simulink model "Eem_StMac_Prj"  (R2013b)
settings: Solver=FixedStepDiscrete  StartTime=0.0  StopTime=inf  FixedStep=0.001  RelTol=1e-3
PreLoadFcn:
  | load('Eem_StMac_Sim_DataSpec.mat')
model workspace (MAT data in the model file):
  cfg_mdx : org.apache.xerces.dom.DocumentImpl (value not decoded)
  cfg_mdx_status = ASAM_PSP.MDX.Config.ConfigStatus
undefined symbols (not defined in the file): process, ProcessTrigger_Lib
libraries: Variable_Lib x21, Efx_Library x17, Parameter_Lib x16, DSM_Library x9, DeltaTime_Lib x2, SYC_Library x1, DGS_Misc_Lib x1
(part 1 of 2)
PreSaveFcn:
  | %BOSCHToolsStart
  | if exist('saveWorkspaceToMatFile','file')
  | saveWorkspaceToMatFile(bdroot);
  | end;
  | %BOSCHToolsEnd
settings Model: NumberOfSteps=100  Creator=gjg2si  LastModifiedBy=bij2si
settings DataIOCC: SaveFormat=StructureWithTime  SignalLoggingSaveFormat=ModelDataLogs  SaveOutput=off  SignalLogging=off  DSMLogging=off  SaveTime=off
settings OptimizationCC: InlineParams=on  UseIntDivNetSlope=on  UseFloatMulNetSlope=on  DefaultUnderspecifiedDataType=single  InlineInvariantSignals=on  EnhancedBackFolding=on  StrengthReduction=on  EnableMemcpy=off  PassReuseOutputArgsAs=Individual arguments  ExpressionDepthLimit=2147483647  ZeroExternalMemoryAtStartup=off  ZeroInternalMemoryAtStartup=off  InitFltsAndDblsToZero=on  EfficientFloat2IntCast=on  OptimizeModelRefInitCode=on  SimCompilerOptimization=On  AccelVerboseBuild=on
settings DebuggingCC: ConsistencyChecking=error  SignalInfNanChecking=warning  SignalRangeChecking=error  AlgebraicLoopMsg=error  UnderspecifiedInitializationDetection=Simplified  BlockPriorityViolationMsg=error  MinStepSizeMsg=error  SolverPrmCheckMsg=error  InheritedTsInSrcMsg=none  DiscreteInheritContinuousMsg=error  MultiTaskDSMMsg=warning  TasksWithSamePriorityMsg=error  SigSpecEnsureSampleTimeMsg=error  CheckMatrixSingularityMsg=error  ParameterUnderflowMsg=error  ParameterTunabilityLossMsg=error  FixptConstUnderflowMsg=error  FixptConstOverflowMsg=error  FixptConstPrecisionLossMsg=warning  UnnecessaryDatatypeConvMsg=warning  VectorMatrixConversionMsg=error  SignalLabelMismatchMsg=warning  UnconnectedLineMsg=error  SFcnCompatibilityMsg=warning  UniqueDataStoreMsg=error  RootOutportRequireBusObject=error  ModelReferenceIOMsg=error  ModelReferenceVersionMismatchMessage=warning  ModelReferenceIOMismatchMessage=warning  UnknownTsInhSupMsg=error  StateNameClashWarn=warning  SimStateInterfaceChecksumMismatchMsg=error  StrictBusMsg=ErrorOnBusTreatedAsVector  BusNameAdapt=ErrorWithoutRepair  NonBusSignalsTreatedAsBus=error  SFUnexpectedBacktrackingDiag=error  SFInvalidInputDataAccessInChartInitDiag=error  SFNoUnconditionalDefaultTransitionDiag=error  SFUnconditionalTransitionShadowingDiag=error
settings HardwareCC: ProdIntDivRoundTo=Zero  ProdHWDeviceType=Generic->32-bit Embedded Processor
settings ModelReferenceCC: ModelReferenceNumInstancesAllowed=Single
settings RTWCC: SystemTargetFile=mdxtarget.tlc  GenCodeOnly=on  GenerateMakefile=off  TemplateMakefile=mdxtarget.tmf  Description=Bosch MDX Target  GenerateReport=on  ProcessScript=mdxtarget_make_rtw_hook  IncludeHyperlinkInReport=on  LaunchReport=on  GenerateTraceInfo=on  GenerateTraceReport=on  GenerateTraceReportSl=on  GenerateTraceReportSf=on  GenerateTraceReportEml=on  RTWCompilerOptimization=On
settings CodeAppCC: ForceParamTrailComments=on  IgnoreCustomStorageClasses=off  IgnoreTestpoints=on  MaxIdLength=60  SFDataObjDesc=on  MangleLength=3  CustomSymbolStrField=$N$M_$A  CustomSymbolStrFcnArg=arg$I$N$M  CustomSymbolStrBlkIO=_tb_$A_$M  CustomSymbolStrTmpVar=_t_$A_$M  InsertBlockDesc=on  MATLABSourceComments=on
settings STFCustomTargetCC: CodeReplacementLibrary=AUTOSAR 4.0  UtilityFuncGeneration=Shared location  ERTMultiwordTypeDef=User defined  ERTMultiwordLength=0  IncludeMdlTerminateFcn=off  CombineOutputUpdateFcns=on  SuppressErrorStatus=on  ERTCustomFileBanners=on  SupportAbsoluteTime=off  SupportNonFinite=off  SupportComplex=off  SupportContinuousTime=off  SupportNonInlinedSFcns=off  ParenthesesLevel=Maximum  MATLABClassNameForMDSCustomization=Simulink.SoftwareTarget.ERTCustomization  GRTInterface=off  SystemTargetFile=mdxtarget.tlc
settings ERTTargetCC: CodeReplacementLibrary=AUTOSAR 4.0  UtilityFuncGeneration=Shared location  ERTMultiwordTypeDef=User defined  ERTMultiwordLength=0  ParMdlRefBuildCompliant=off  CompOptLevelCompliant=off  ConcurrentExecutionCompliant=off  IncludeMdlTerminateFcn=off  SuppressErrorStatus=on  ERTFirstTimeCompliant=off  SupportAbsoluteTime=off  SupportNonFinite=off  SupportComplex=off  ParenthesesLevel=Maximum  ModelStepFunctionPrototypeControlCompliant=off  CPPClassGenCompliant=off  GenerateASAP2=on  InlinedParameterPlacement=NonHierarchical  ERTSrcFileBannerTemplate=bosch_mdx_template.cgt  ERTHdrFileBannerTemplate=bosch_h_template.cgt  ERTCustomFileTemplate=mdx_file_process.tlc  ERTFilePackagingFormat=Compact  PreserveExpressionOrder=on  PreserveIfCondition=on  PreserveExternInFcnDecls=off

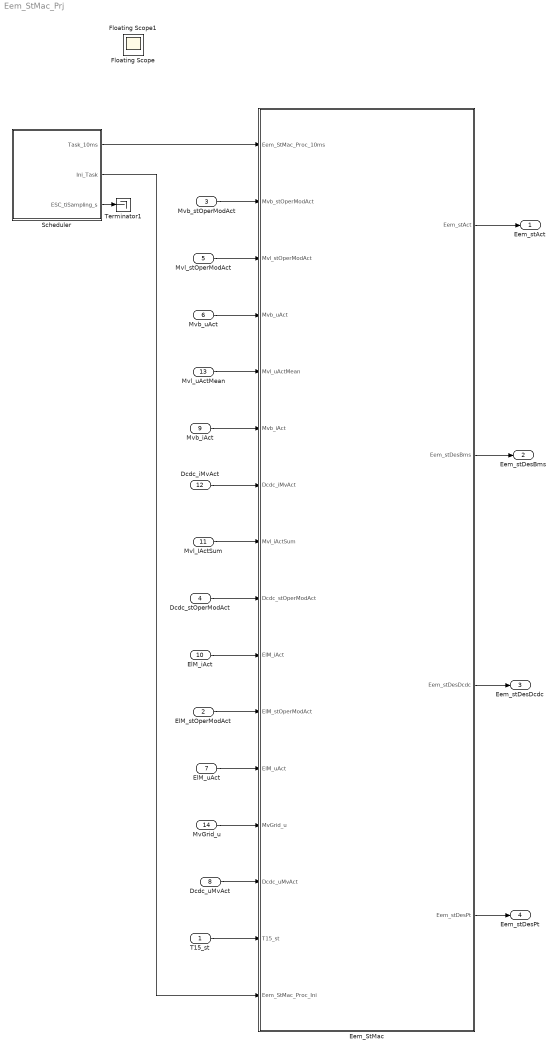
== system Eem_StMac_Prj ==
  T15_st : Inport  OutDataTypeStr=boolean
  ElM_stOperModAct : Inport  Port=2  OutDataTypeStr=OneToOne_U8
  Mvb_stOperModAct : Inport  Port=3  OutDataTypeStr=OneToOne_U8
  Dcdc_stOperModAct : Inport  Port=4  OutDataTypeStr=OneToOne_U8
  Mvl_stOperModAct : Inport  Port=5  OutDataTypeStr=OneToOne_U8
  Mvb_uAct : Inport  Port=6  OutDataTypeStr=spg_q0p0039_S16
  ElM_uAct : Inport  Port=7  OutDataTypeStr=spg_q0p0039_S16
  Dcdc_uMvAct : Inport  Port=8  OutDataTypeStr=spg_q0p0039_S16
  Mvb_iAct : Inport  Port=9  OutDataTypeStr=Curr_A_q0p03125_COMPU_S16
  ElM_iAct : Inport  Port=10  OutDataTypeStr=Curr_A_q0p03125_COMPU_S16
  Mvl_IActSum : Inport  Port=11  OutDataTypeStr=Curr_A_q0p03125_COMPU_S16
  Dcdc_iMvAct : Inport  Port=12  OutDataTypeStr=Curr_A_q0p03125_COMPU_S16
  Mvl_uActMean : Inport  Port=13  OutDataTypeStr=spg_q0p0039_S16
  MvGrid_u : Inport  Port=14  OutDataTypeStr=spg_q0p0039_S16
  Eem_StMac : Subsystem
  Scheduler : Subsystem  mask(Scheduler){Task_1ms=off, Task_2ms=off, Task_5ms=off, Task_10ms=on, Task_20ms=off, Task_50ms=off, Task_100ms=off, Task_200ms=off, Task_1000ms=off, Ini_Task=on, ASync_Task=off}
      mask help:
      | This Scheduler can be used to simulate execution of different
      | runnables/processes. Needed tasks can be de-/activated by this mask.
      |
      | Beside different time rates there is one task for initialization and
      | an asynchonous task that is triggered depending on ASync_U.
      mask init:
      | scheduler_cb('Ini',gcs,gcb);
  Terminator1 : Terminator
  Eem_stAct : Outport  OutDataTypeStr=OneToOne_U16
  Eem_stDesBms : Outport  Port=2  OutDataTypeStr=OneToOne_U8
  Eem_stDesDcdc : Outport  Port=3  OutDataTypeStr=OneToOne_U8
  Eem_stDesPt : Outport  Port=4  OutDataTypeStr=OneToOne_U8
  Floating Scope : Scope
      settings: Floating=on  YMin=0  YMax=700
  Floating Scope1 : Scope
      settings: Floating=on  YMin=0  YMax=2000
  wires:
  Scheduler/3(ESC_tiSampling_s) -> Terminator1/1
  Mvb_stOperModAct/1 -> Eem_StMac/2(Mvb_stOperModAct)
  Dcdc_stOperModAct/1 -> Eem_StMac/9(Dcdc_stOperModAct)
  Mvb_uAct/1 -> Eem_StMac/4(Mvb_uAct)
  Mvl_uActMean/1 -> Eem_StMac/5(Mvl_uActMean)
  Mvb_iAct/1 -> Eem_StMac/6(Mvb_iAct)
  Dcdc_iMvAct/1 -> Eem_StMac/7(Dcdc_iMvAct)
  Mvl_IActSum/1 -> Eem_StMac/8(Mvl_iActSum)
  Eem_StMac/1(Eem_stAct) -> Eem_stAct/1
  Eem_StMac/2(Eem_stDesBms) -> Eem_stDesBms/1
  Eem_StMac/4(Eem_stDesPt) -> Eem_stDesPt/1
  Eem_StMac/3(Eem_stDesDcdc) -> Eem_stDesDcdc/1
  Mvl_stOperModAct/1 -> Eem_StMac/3(Mvl_stOperModAct)
  Scheduler/1(Task_10ms) -> Eem_StMac/1(Eem_StMac_Proc_10ms)
  ElM_stOperModAct/1 -> Eem_StMac/11(ElM_stOperModAct)
  ElM_iAct/1 -> Eem_StMac/10(ElM_iAct)
  ElM_uAct/1 -> Eem_StMac/12(ElM_uAct)
  MvGrid_u/1 -> Eem_StMac/13(MvGrid_u)
  T15_st/1 -> Eem_StMac/15(T15_st)
  Dcdc_uMvAct/1 -> Eem_StMac/14(Dcdc_uMvAct)
  Scheduler/2(Ini_Task) -> Eem_StMac/16(Eem_StMac_Proc_Ini)

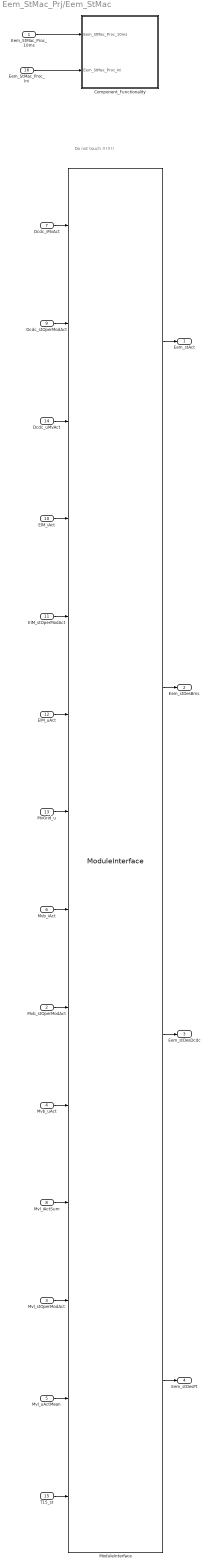
== system Eem_StMac_Prj/Eem_StMac ==
  note: Do not touch !!!!!!!
  Eem_StMac_Proc_10ms : Inport
  Mvb_stOperModAct : Inport  Port=2
  Mvl_stOperModAct : Inport  Port=3
  Mvb_uAct : Inport  Port=4
  Mvl_uActMean : Inport  Port=5
  Mvb_iAct : Inport  Port=6
  Dcdc_iMvAct : Inport  Port=7
  Mvl_iActSum : Inport  Port=8
  Dcdc_stOperModAct : Inport  Port=9
  ElM_iAct : Inport  Port=10
  ElM_stOperModAct : Inport  Port=11
  ElM_uAct : Inport  Port=12
  MvGrid_u : Inport  Port=13
  Dcdc_uMvAct : Inport  Port=14
  T15_st : Inport  Port=15
  Eem_StMac_Proc_Ini : Inport  Port=16
  Component_Functionality : Subsystem
  ModuleInterface : DGS_Misc_Lib/ModuleInterface
      link override FromIRV_OutIrv1: GotoTag=IRV_OutIrv1
      link override GotoIRV: GotoTag=IRV_InIrv  TagVisibility=global
  Eem_stAct : Outport
  Eem_stDesBms : Outport  Port=2
  Eem_stDesDcdc : Outport  Port=3
  Eem_stDesPt : Outport  Port=4
  wires:
  Eem_StMac_Proc_10ms/1 -> Component_Functionality/1(Eem_StMac_Proc_10ms)
  Eem_StMac_Proc_Ini/1 -> Component_Functionality/2(Eem_StMac_Proc_Ini)
  Dcdc_iMvAct/1 -> ModuleInterface/1
  Dcdc_stOperModAct/1 -> ModuleInterface/2
  Dcdc_uMvAct/1 -> ModuleInterface/3
  ElM_iAct/1 -> ModuleInterface/4
  ElM_stOperModAct/1 -> ModuleInterface/5
  ElM_uAct/1 -> ModuleInterface/6
  MvGrid_u/1 -> ModuleInterface/7
  Mvb_iAct/1 -> ModuleInterface/8
  Mvb_stOperModAct/1 -> ModuleInterface/9
  Mvb_uAct/1 -> ModuleInterface/10
  Mvl_iActSum/1 -> ModuleInterface/11
  Mvl_stOperModAct/1 -> ModuleInterface/12
  Mvl_uActMean/1 -> ModuleInterface/13
  T15_st/1 -> ModuleInterface/14
  ModuleInterface/1 -> Eem_stAct/1
  ModuleInterface/2 -> Eem_stDesBms/1
  ModuleInterface/3 -> Eem_stDesDcdc/1
  ModuleInterface/4 -> Eem_stDesPt/1

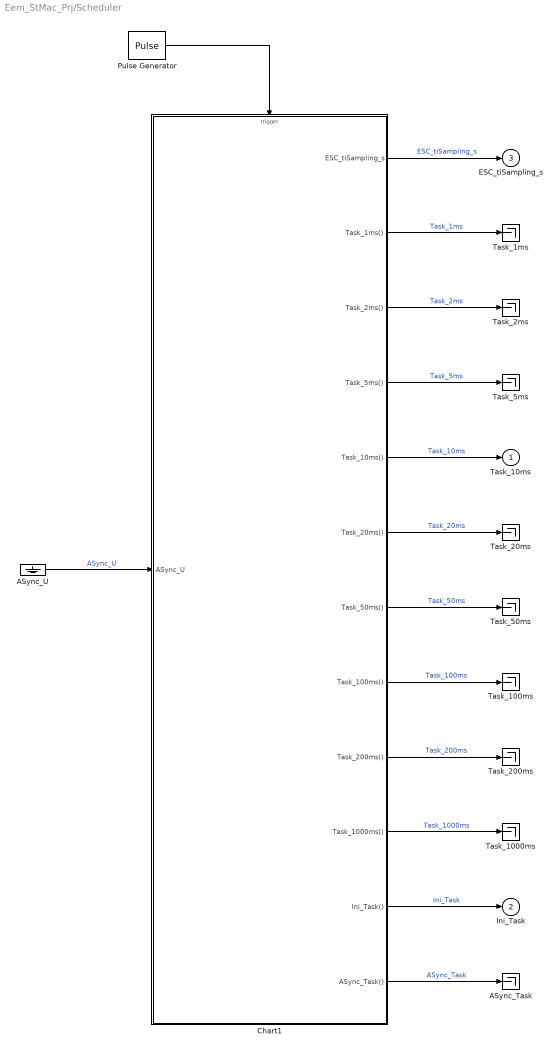
== system Eem_StMac_Prj/Scheduler ==
  ASync_Task : Terminator
  ASync_U : Ground
  Chart1 : Stateflow chart  TreatAsAtomicUnit=on  SystemSampleTime=0.001
  Pulse Generator : DiscretePulseGenerator  SampleTime=.001
  Task_1000ms : Terminator
  Task_100ms : Terminator
  Task_1ms : Terminator
  Task_200ms : Terminator
  Task_20ms : Terminator
  Task_2ms : Terminator
  Task_50ms : Terminator
  Task_5ms : Terminator
  Task_10ms : Outport  PortDimensions=1  LockScale=on
  Ini_Task : Outport  Port=2  PortDimensions=1  LockScale=on
  ESC_tiSampling_s : Outport  Port=3  PortDimensions=1  LockScale=on
  wires:
  Chart1/1(ESC_tiSampling_s) -> ESC_tiSampling_s/1  "ESC_tiSampling_s"
  Pulse Generator/1 -> Chart1/Trigger
  Chart1/12(ASync_Task()) -> ASync_Task/1  "ASync_Task"
  Chart1/11(Ini_Task()) -> Ini_Task/1  "Ini_Task"
  Chart1/10(Task_1000ms()) -> Task_1000ms/1  "Task_1000ms"
  Chart1/9(Task_200ms()) -> Task_200ms/1  "Task_200ms"
  Chart1/8(Task_100ms()) -> Task_100ms/1  "Task_100ms"
  Chart1/7(Task_50ms()) -> Task_50ms/1  "Task_50ms"
  Chart1/6(Task_20ms()) -> Task_20ms/1  "Task_20ms"
  Chart1/5(Task_10ms()) -> Task_10ms/1  "Task_10ms"
  Chart1/4(Task_5ms()) -> Task_5ms/1  "Task_5ms"
  Chart1/3(Task_2ms()) -> Task_2ms/1  "Task_2ms"
  Chart1/2(Task_1ms()) -> Task_1ms/1  "Task_1ms"
  ASync_U/1 -> Chart1/1(ASync_U)  "ASync_U"

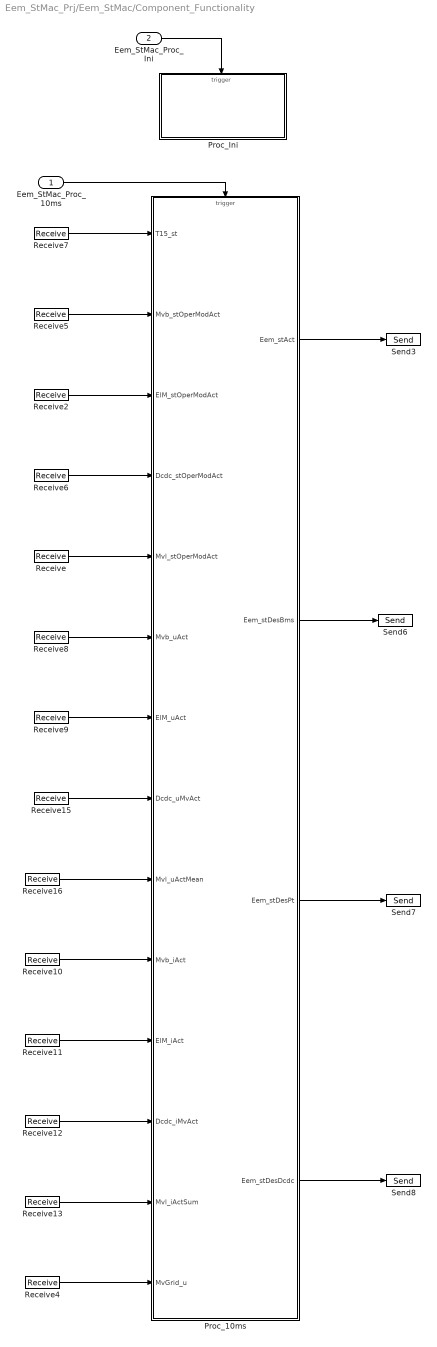
== system Eem_StMac_Prj/Eem_StMac/Component_Functionality ==
  Eem_StMac_Proc_10ms : Inport
  Eem_StMac_Proc_Ini : Inport  Port=2
  Proc_10ms : Subsystem  TreatAsAtomicUnit=on
  Proc_Ini : Subsystem  TreatAsAtomicUnit=on
  Receive : Variable_Lib/Receive  Description=Receive block  Par_Signal=Mvl_stOperModAct  Par_Dim=1  Par_Dt=OneToOne_U8  Par_SignalOld=Mvl_stOperModAct  Par_Scope=Global  Par_Addr=FastNoReIni
      settings: AttributesFormatString=Mvl_stOperModAct
  Receive10 : Variable_Lib/Receive  Description=Receive block  Par_Signal=Mvb_iAct  Par_Dim=1  Par_Dt=Curr_A_q0p03125_COMPU_S16  Par_SignalOld=Mvb_iAct  Par_Scope=Global  Par_Addr=FastNoReIni
      settings: AttributesFormatString=Mvb_iAct
  Receive11 : Variable_Lib/Receive  Description=Receive block  Par_Signal=ElM_iAct  Par_Dim=1  Par_Dt=Curr_A_q0p03125_COMPU_S16  Par_SignalOld=ElM_iAct  Par_Scope=Global  Par_Addr=FastNoReIni
      settings: AttributesFormatString=ElM_iAct
  Receive12 : Variable_Lib/Receive  Description=Receive block  Par_Signal=Dcdc_iMvAct  Par_Dim=1  Par_Dt=Curr_A_q0p03125_COMPU_S16  Par_SignalOld=Dcdc_iMvAct  Par_Scope=Global  Par_Addr=FastNoReIni
      settings: AttributesFormatString=Dcdc_iMvAct
  Receive13 : Variable_Lib/Receive  Description=Receive block  Par_Signal=Mvl_iActSum  Par_Dim=1  Par_Dt=Curr_A_q0p03125_COMPU_S16  Par_SignalOld=Mvl_iActSum  Par_Scope=Global  Par_Addr=FastNoReIni
      settings: AttributesFormatString=Mvl_iActSum
  Receive15 : Variable_Lib/Receive  Description=Receive block  Par_Signal=Dcdc_uMvAct  Par_Dim=1  Par_Dt=spg_q0p0039_S16  Par_SignalOld=Dcdc_uMvAct  Par_Scope=Global  Par_Addr=FastNoReIni
      settings: AttributesFormatString=Dcdc_uMvAct
  Receive16 : Variable_Lib/Receive  Description=Receive block  Par_Signal=Mvl_uActMean  Par_Dim=1  Par_Dt=spg_q0p0039_S16  Par_SignalOld=Mvl_uActMean  Par_Scope=Global  Par_Addr=FastNoReIni
      settings: AttributesFormatString=Mvl_uActMean
  Receive2 : Variable_Lib/Receive  Description=Receive block  Par_Signal=ElM_stOperModAct  Par_Dim=1  Par_Dt=OneToOne_U8  Par_SignalOld=ElM_stOperModAct  Par_Scope=Global  Par_Addr=FastNoReIni
      settings: AttributesFormatString=ElM_stOperModAct
  Receive4 : Variable_Lib/Receive  Description=Receive block  Par_Signal=MvGrid_u  Par_Dim=1  Par_Dt=spg_q0p0039_S16  Par_SignalOld=MvGrid_u  Par_Scope=Global  Par_Addr=FastNoReIni
      settings: AttributesFormatString=MvGrid_u
  Receive5 : Variable_Lib/Receive  Description=Receive block  Par_Signal=Mvb_stOperModAct  Par_Dim=1  Par_Dt=OneToOne_U8  Par_SignalOld=Mvb_stOperModAct  Par_Scope=Global  Par_Addr=FastNoReIni
      settings: AttributesFormatString=Mvb_stOperModAct
  Receive6 : Variable_Lib/Receive  Description=Receive block  Par_Signal=Dcdc_stOperModAct  Par_Dim=1  Par_Dt=OneToOne_U8  Par_SignalOld=Dcdc_stOperModAct  Par_Scope=Global  Par_Addr=FastNoReIni
      settings: AttributesFormatString=Dcdc_stOperModAct
  Receive7 : Variable_Lib/Receive  Description=Receive block  Par_Signal=T15_st  Par_Dim=1  Par_Dt=boolean  Par_SignalOld=T15_st  Par_Scope=Global  Par_Addr=FastNoReIni
      settings: AttributesFormatString=T15_st
  Receive8 : Variable_Lib/Receive  Description=Receive block  Par_Signal=Mvb_uAct  Par_Dim=1  Par_Dt=spg_q0p0039_S16  Par_SignalOld=Mvb_uAct  Par_Scope=Global  Par_Addr=FastNoReIni
      settings: AttributesFormatString=Mvb_uAct
  Receive9 : Variable_Lib/Receive  Description=Receive block  Par_Signal=ElM_uAct  Par_Dim=1  Par_Dt=spg_q0p0039_S16  Par_SignalOld=ElM_uAct  Par_Scope=Global  Par_Addr=FastNoReIni
      settings: AttributesFormatString=ElM_uAct
  Send3 : Variable_Lib/Send  Description=Send block  Par_Signal=Eem_stAct  Par_Dim=1  Par_Dt=OneToOne_U16  Par_Access=Write  Par_SignalOld=Eem_stAct  Par_Scope=Global  Par_Addr=FastNoReIni
      settings: AttributesFormatString=Eem_stAct
  Send6 : Variable_Lib/Send  Description=Send block  Par_Signal=Eem_stDesBms  Par_Dim=1  Par_Dt=OneToOne_U8  Par_Access=Write  Par_SignalOld=Eem_stDesBms  Par_Scope=Global  Par_Addr=FastNoReIni
      settings: AttributesFormatString=Eem_stDesBms
  Send7 : Variable_Lib/Send  Description=Send block  Par_Signal=Eem_stDesPt  Par_Dim=1  Par_Dt=OneToOne_U8  Par_Access=Write  Par_SignalOld=Eem_stDesPt  Par_Scope=Global  Par_Addr=FastNoReIni
      settings: AttributesFormatString=Eem_stDesPt
  Send8 : Variable_Lib/Send  Description=Send block  Par_Signal=Eem_stDesDcdc  Par_Dim=1  Par_Dt=OneToOne_U8  Par_Access=Write  Par_SignalOld=Eem_stDesDcdc  Par_Scope=Global  Par_Addr=FastNoReIni
      settings: AttributesFormatString=Eem_stDesDcdc
  wires:
  Eem_StMac_Proc_10ms/1 -> Proc_10ms/Trigger
  Receive13/1 -> Proc_10ms/13(Mvl_iActSum)
  Receive12/1 -> Proc_10ms/12(Dcdc_iMvAct)
  Receive11/1 -> Proc_10ms/11(ElM_iAct)
  Receive10/1 -> Proc_10ms/10(Mvb_iAct)
  Receive16/1 -> Proc_10ms/9(Mvl_uActMean)
  Receive15/1 -> Proc_10ms/8(Dcdc_uMvAct)
  Receive9/1 -> Proc_10ms/7(ElM_uAct)
  Receive8/1 -> Proc_10ms/6(Mvb_uAct)
  Receive/1 -> Proc_10ms/5(Mvl_stOperModAct)
  Receive6/1 -> Proc_10ms/4(Dcdc_stOperModAct)
  Receive2/1 -> Proc_10ms/3(ElM_stOperModAct)
  Receive5/1 -> Proc_10ms/2(Mvb_stOperModAct)
  Proc_10ms/1(Eem_stAct) -> Send3/1
  Proc_10ms/2(Eem_stDesBms) -> Send6/1
  Proc_10ms/3(Eem_stDesPt) -> Send7/1
  Proc_10ms/4(Eem_stDesDcdc) -> Send8/1
  Receive7/1 -> Proc_10ms/1(T15_st)
  Receive4/1 -> Proc_10ms/14(MvGrid_u)
  Eem_StMac_Proc_Ini/1 -> Proc_Ini/Trigger

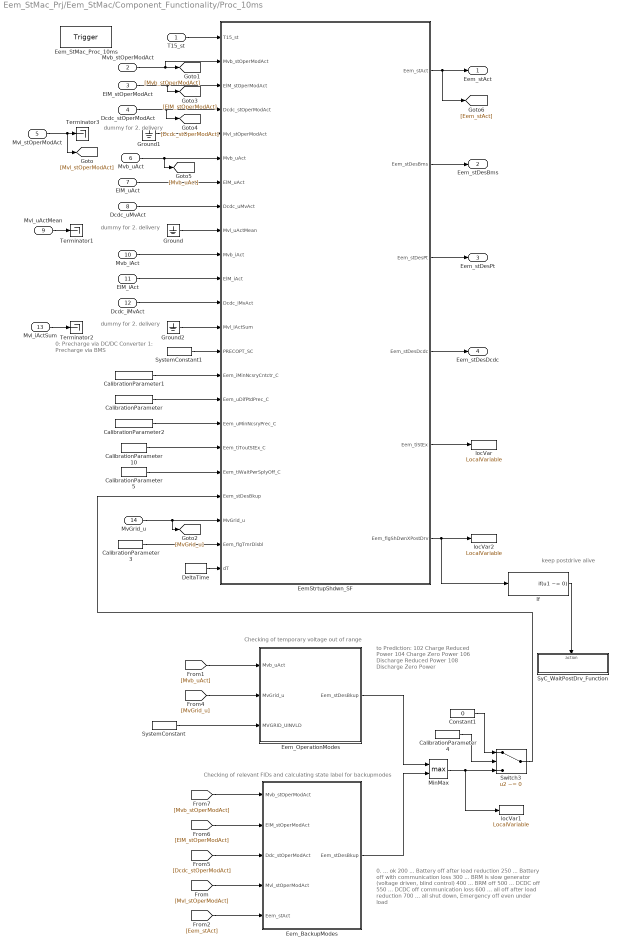
== system Eem_StMac_Prj/Eem_StMac/Component_Functionality/Proc_10ms ==
  note: keep postdrive alive
  note: Checking of temporary voltage out of range
  note: Checking of relevant FIDs and calculating state label for backupmodes
  note: 0: Precharge via DC/DC Converter
      | 1: Precharge via BMS
  note: 0.            ...  ok
      | 200 ... Battery off after load reduction
      | 250 ... Battery off with communication loss
      | 300 ... BRM is slow generator (voltage driven, blind control)
      | 400 ... BRM off
      | 500 ... DCDC off
      | 550 ... DCDC off communication loss
      | 600 ... all off after load reduction
      | 700 ... all shut down, Emergency off even under load
  note: to Prediction:
      | 102  Charge Reduced Power
      | 104  Charge Zero Power
      | 106  Discharge Reduced Power
      | 108  Discharge Zero Power
  note: dummy for
      | 2. delivery
  note: dummy for
      | 2. delivery
  note: dummy for
      | 2. delivery
  T15_st : Inport
  Mvb_stOperModAct : Inport  Port=2
  ElM_stOperModAct : Inport  Port=3
  Dcdc_stOperModAct : Inport  Port=4
  Mvl_stOperModAct : Inport  Port=5
  Mvb_uAct : Inport  Port=6
  ElM_uAct : Inport  Port=7
  Dcdc_uMvAct : Inport  Port=8
  Mvl_uActMean : Inport  Port=9
  Mvb_iAct : Inport  Port=10
  ElM_iAct : Inport  Port=11
  Dcdc_iMvAct : Inport  Port=12
  Mvl_iActSum : Inport  Port=13
  MvGrid_u : Inport  Port=14  OutDataTypeStr=spg_q0p0039_S16
  Eem_StMac_Proc_10ms : TriggerPort  LibraryBlock=ProcessTrigger_Lib/process  procName=Eem_StMac_Proc_10ms
      settings: AttributesFormatString=Process: %<procName>
  CalibrationParameter : Parameter_Lib/CalibrationParameter  ParName=Eem_uDifPtdPrec_C  ParVal=5  ParValStruct=<1x1 struct>  ParValDt=spg_q0p0039_S16  Par_MDX=off  ParNameOld=Eem_uDifPtdPrec_C  Value=0  Par_Name=0
      settings: AttributesFormatString=%<ParName>
  CalibrationParameter1 : Parameter_Lib/CalibrationParameter  ParName=Eem_iMinNcsryCntctr_C  ParVal=3  ParValStruct=<1x1 struct>  ParValDt=Curr_A_q0p03125_COMPU_S16  Par_MDX=off  ParNameOld=Eem_iMinNcsryCntctr_C  Value=0  Par_Name=0
      settings: AttributesFormatString=%<ParName>
  CalibrationParameter10 : Parameter_Lib/CalibrationParameter  ParName=Eem_tiToutStEx_C  ParVal=10  ParValStruct=<1x1 struct>  ParValDt=RBPtCel_ti_0p01_1_U16  Par_MDX=off  ParNameOld=Eem_tiToutStEx_C  Value=0  Par_Name=0
      settings: AttributesFormatString=%<ParName>
  CalibrationParameter2 : Parameter_Lib/CalibrationParameter  ParName=Eem_uMinNcsryPrec_C  ParVal=30  ParValStruct=<1x1 struct>  ParValDt=spg_q0p0039_S16  Par_MDX=off  ParNameOld=Eem_uMinNcsryPrec_C  Value=0  Par_Name=0
      settings: AttributesFormatString=%<ParName>
  CalibrationParameter3 : Parameter_Lib/CalibrationParameter  ParName=Eem_flgTmrDisbl_C  ParVal=0  ParValStruct=<1x1 struct>  ParValDt=boolean  Par_MDX=off  ParNameOld=Eem_flgTmrDisbl_C  Value=0  Par_Name=0
      settings: AttributesFormatString=%<ParName>
  CalibrationParameter4 : Parameter_Lib/CalibrationParameter  ParName=Eem_flgBkupDisbl_C  ParVal=0  ParValStruct=<1x1 struct>  ParValDt=boolean  Par_MDX=off  ParNameOld=Eem_flgBkupDisbl_C  Value=0  Par_Name=0
      settings: AttributesFormatString=%<ParName>
  CalibrationParameter5 : Parameter_Lib/CalibrationParameter  ParName=Eem_tiWaitPwrSplyOff_C  ParVal=2  ParValStruct=<1x1 struct>  ParValDt=RBPtCel_ti_0p01_1_U16  Par_MDX=off  ParNameOld=Eem_tiWaitPwrSplyOff_C  Value=0  Par_Name=0
      settings: AttributesFormatString=%<ParName>
  Constant1 : Constant  Value=0  OutDataTypeStr=OneToOne_U16
  DeltaTime : DeltaTime_Lib/DeltaTime  outDType=sfix32_S1en6  initVal=.01
  EemStrtupShdwn_SF : Stateflow chart  TreatAsAtomicUnit=on
      settings: MinAlgLoopOccurrences=on
  Eem_BackupModes : Subsystem
  Eem_OperationModes : Subsystem
  Ground : Ground
  Ground1 : Ground
  Ground2 : Ground
  If : If  IfExpression=u1 ~= 0  ShowElse=off
  MinMax : MinMax  Function=max  Inputs=2  OutDataTypeStr=OneToOne_U16  RndMeth=Simplest  SaturateOnIntegerOverflow=on
  Switch3 : Switch  Criteria=u2 ~= 0  RndMeth=Simplest  SaturateOnIntegerOverflow=on
      settings: AttributesFormatString=%<Criteria>\nThreshold:%<Threshold>
  SyC_WaitPostDrv_Function : Subsystem  TreatAsAtomicUnit=on
  SystemConstant : Parameter_Lib/SystemConstant  ParName=MVGRID_UINVLD  ParVal=0  ParValDt=spg_q0p0039_S16  Par_MDX=off  ParNameOld=MVGRID_UINVLD  Par_Name=0
      settings: AttributesFormatString=%<ParName>
  SystemConstant1 : Parameter_Lib/SystemConstant  ParName=PRECOPT_SC  ParVal=0  ParValDt=OneToOne_U8  Par_MDX=off  ParNameOld=PRECOPT_SC  Par_Name=0
      settings: AttributesFormatString=%<ParName>
  Terminator1 : Terminator
  Terminator2 : Terminator
  Terminator3 : Terminator
  locVar : Variable_Lib/LocalVariable  Description=locVar block  Par_Signal=Eem_tiStEx  Par_Dim=1  Par_Dt=RBPtCel_ti_0p01_1_U16  Par_Access=Write  Par_Enable=off  Par_MultipleInstance=on  Par_SignalOld=Eem_tiStEx  Par_Addr=FastNoReIni
      settings: AttributesFormatString=Eem_tiStEx
  locVar1 : Variable_Lib/LocalVariable  Description=locVar block  Par_Signal=Eem_stDesBkup  Par_Dim=1  Par_Dt=OneToOne_U16  Par_Access=Write  Par_Enable=off  Par_MultipleInstance=on  Par_SignalOld=Eem_stDesBkup  Par_Addr=FastNoReIni
      settings: AttributesFormatString=Eem_stDesBkup
  locVar2 : Variable_Lib/LocalVariable  Description=locVar block  Par_Signal=Eem_flgShDwnXPostDrv  Par_Dim=1  Par_Dt=boolean  Par_Access=ReadWrite  Par_Enable=off  Par_MultipleInstance=off  Par_SignalOld=Eem_flgShDwnXPostDrv  Par_Addr=FastNoReIni
      settings: AttributesFormatString=Eem_flgShDwnXPostDrv
  Eem_stAct : Outport  OutDataTypeStr=OneToOne_U16
  Eem_stDesBms : Outport  Port=2
  Eem_stDesPt : Outport  Port=3
  Eem_stDesDcdc : Outport  Port=4
  wires:
  Mvb_uAct/1 -> [Mvb_uAct], EemStrtupShdwn_SF/6(Mvb_uAct)
  ElM_uAct/1 -> EemStrtupShdwn_SF/7(ElM_uAct)
  ElM_stOperModAct/1 -> [ElM_stOperModAct], EemStrtupShdwn_SF/3(ElM_stOperModAct)
  Dcdc_stOperModAct/1 -> [Dcdc_stOperModAct], EemStrtupShdwn_SF/4(Dcdc_stOperModAct)
  Dcdc_uMvAct/1 -> EemStrtupShdwn_SF/8(Dcdc_uMvAct)
  Mvb_iAct/1 -> EemStrtupShdwn_SF/10(Mvb_iAct)
  EemStrtupShdwn_SF/2(Eem_stDesBms) -> Eem_stDesBms/1
  EemStrtupShdwn_SF/3(Eem_stDesPt) -> Eem_stDesPt/1
  EemStrtupShdwn_SF/4(Eem_stDesDcdc) -> Eem_stDesDcdc/1
  Mvb_stOperModAct/1 -> [Mvb_stOperModAct], EemStrtupShdwn_SF/2(Mvb_stOperModAct)
  ElM_iAct/1 -> EemStrtupShdwn_SF/11(ElM_iAct)
  Dcdc_iMvAct/1 -> EemStrtupShdwn_SF/12(Dcdc_iMvAct)
  SystemConstant1/1 -> EemStrtupShdwn_SF/14(PRECOPT_SC)
  CalibrationParameter1/1 -> EemStrtupShdwn_SF/15(Eem_iMinNcsryCntctr_C)
  CalibrationParameter/1 -> EemStrtupShdwn_SF/16(Eem_uDifPtdPrec_C)
  CalibrationParameter2/1 -> EemStrtupShdwn_SF/17(Eem_uMinNcsryPrec_C)
  Eem_OperationModes/1(Eem_stDesBkup) -> MinMax/1
  Eem_BackupModes/1(Eem_stDesBkup) -> MinMax/2
  CalibrationParameter10/1 -> EemStrtupShdwn_SF/18(Eem_tiToutStEx_C)
  Mvl_stOperModAct/1 -> [Mvl_stOperModAct], Terminator3/1
  [Mvl_stOperModAct] -> Eem_BackupModes/4(Mvl_stOperModAct)
  T15_st/1 -> EemStrtupShdwn_SF/1(T15_st)
  [Mvb_uAct] -> Eem_OperationModes/1(Mvb_uAct)
  [Mvb_stOperModAct] -> Eem_BackupModes/1(Mvb_stOperModAct)
  [ElM_stOperModAct] -> Eem_BackupModes/2(ElM_stOperModAct)
  [Dcdc_stOperModAct] -> Eem_BackupModes/3(Ddc_stOperModAct)
  DeltaTime/1 -> EemStrtupShdwn_SF/23(dT)
  If/1 -> SyC_WaitPostDrv_Function/Action
  SystemConstant/1 -> Eem_OperationModes/3(MVGRID_UINVLD)
  [MvGrid_u] -> Eem_OperationModes/2(MvGrid_u)
  MvGrid_u/1 -> [MvGrid_u], EemStrtupShdwn_SF/21(MvGrid_u)
  Mvl_uActMean/1 -> Terminator1/1
  Mvl_iActSum/1 -> Terminator2/1
  CalibrationParameter3/1 -> EemStrtupShdwn_SF/22(Eem_flgTmrDisbl)
  EemStrtupShdwn_SF/5(Eem_tiStEx) -> locVar/1
  Ground/1 -> EemStrtupShdwn_SF/9(Mvl_uActMean)
  Ground1/1 -> EemStrtupShdwn_SF/5(Mvl_stOperModAct)
  Ground2/1 -> EemStrtupShdwn_SF/13(Mvl_iActSum)
  Constant1/1 -> Switch3/1
  Switch3/1 -> EemStrtupShdwn_SF/20(Eem_stDesBkup)
  MinMax/1 -> locVar1/1, Switch3/3
  CalibrationParameter4/1 -> Switch3/2
  EemStrtupShdwn_SF/6(Eem_flgShDwnXPostDrv) -> locVar2/1, If/1
  CalibrationParameter5/1 -> EemStrtupShdwn_SF/19(Eem_tiWaitPwrSplyOff_C)
  EemStrtupShdwn_SF/1(Eem_stAct) -> [Eem_stAct], Eem_stAct/1
  [Eem_stAct] -> Eem_BackupModes/5(Eem_stAct)

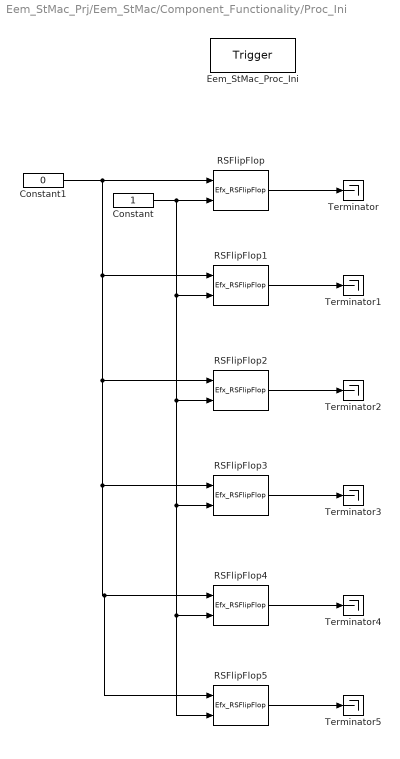
== system Eem_StMac_Prj/Eem_StMac/Component_Functionality/Proc_Ini ==
  Eem_StMac_Proc_Ini : TriggerPort  LibraryBlock=ProcessTrigger_Lib/process  procName=Eem_StMac_Proc_Ini
      settings: AttributesFormatString=Process: %<procName>
  Constant : Constant  OutDataTypeStr=boolean
  Constant1 : Constant  Value=0  OutDataTypeStr=boolean
  RSFlipFlop : Efx_Library/Efx_RSFlipFlop  Par_state=Eem_RSFlipFlop550  Par_StateOld=Eem_RSFlipFlop550
      settings: AttributesFormatString=%<Par_State>
  RSFlipFlop1 : Efx_Library/Efx_RSFlipFlop  Par_state=Eem_RSFlipFlop500  Par_StateOld=Eem_RSFlipFlop500
      settings: AttributesFormatString=%<Par_State>
  RSFlipFlop2 : Efx_Library/Efx_RSFlipFlop  Par_state=Eem_RSFlipFlop400  Par_StateOld=Eem_RSFlipFlop400
      settings: AttributesFormatString=%<Par_State>
  RSFlipFlop3 : Efx_Library/Efx_RSFlipFlop  Par_state=Eem_RSFlipFlop300  Par_StateOld=Eem_RSFlipFlop300
      settings: AttributesFormatString=%<Par_State>
  RSFlipFlop4 : Efx_Library/Efx_RSFlipFlop  Par_state=Eem_RSFlipFlop250  Par_StateOld=Eem_RSFlipFlop250
      settings: AttributesFormatString=%<Par_State>
  RSFlipFlop5 : Efx_Library/Efx_RSFlipFlop  Par_state=Eem_RSFlipFlop200  Par_StateOld=Eem_RSFlipFlop200
      settings: AttributesFormatString=%<Par_State>
  Terminator{,1..5} (6 alike) : Terminator
  wires:
  Constant/1 -> RSFlipFlop1/1, RSFlipFlop5/1, RSFlipFlop4/1, RSFlipFlop3/1, RSFlipFlop2/1, RSFlipFlop/1
  Constant1/1 -> RSFlipFlop5/2, RSFlipFlop4/2, RSFlipFlop3/2, RSFlipFlop2/2, RSFlipFlop1/2, RSFlipFlop/2
  RSFlipFlop/1 -> Terminator/1
  RSFlipFlop1/1 -> Terminator1/1
  RSFlipFlop2/1 -> Terminator2/1
  RSFlipFlop3/1 -> Terminator3/1
  RSFlipFlop4/1 -> Terminator4/1
  RSFlipFlop5/1 -> Terminator5/1

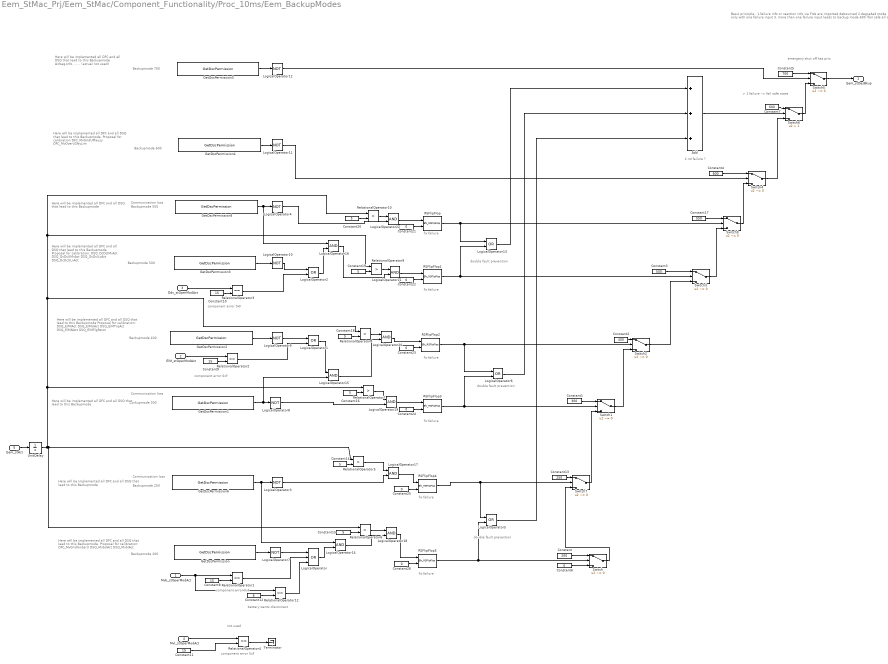
== system Eem_StMac_Prj/Eem_StMac/Component_Functionality/Proc_10ms/Eem_BackupModes ==
  note: Communication loss
  note: not used
  note: component error 0xF
  note: Basic principle :
      | 1.failure info or reaction info via FIds are imported debounced
      | 2.degraded mode only with one failure input
      | 3. more than one failure input leads to backup mode 600 (fail safe all off)
  note: Backupmode 200
  note: Backupmode 300
  note: Backupmode 400
  note: Backupmode 500
  note: Backupmode 600
  note: Backupmode 700
  note: component error 0xF
  note: component error 0xF
  note: component error 0xF
  note: Here will be implemented all DFC and
      | all DSQ that lead to this Backupmode
      | Proposal for calibration:
      |
      |   DSQ_DcDcIMvAct
      |   DSQ_DcDcUMvAct
      |   DSQ_DcDcILvAct
      |   DSQ_DcDcULvAct
  note: Here will be implemented all DFC and all
      | DSQ that lead to this Backupmode.
      | Proposal for calibration
      |
      | DFC_MvGridUPlausy
      | DFC_MvOverUSftyLim
  note: Here will be implemented all DFC and
      | all DSQ that lead to this Backupmode
      |
      | Airbag-Info, ......
      | (actual not used)
  note: Here will be implemented all DFC and all DSQ
      | that lead to this Backupmode
      | Proposal for calibration:
      |
      |   DSQ_ElMIAct
      |   DSQ_ElMUAct
      |   DSQ_ElMTrqAct
      |   DSQ_ElMNAct
      |   DSQ_ElMFlgRstcn
  note: Here will be implemented all DFC and all DSQ
      | that lead to this Backupmode.
      | Proposal for calibration:
      |
      |   DFC_MvGridUnderU
      |
      |   DSQ_MvbUAct
      |   DSQ_MvbIAct
  note: Here will be implemented all DFC and all DSQ
      | that lead to this Backupmode
  note: Backupmode 250
  note: Here will be implemented all DFC and all DSQ
      | that lead to this Backupmode
  note: Backupmode 550
  note: Here will be implemented all DFC and all
      | DSQ that lead to this Backupmode
  note: Communication loss
  note: battery wants disconnect
  note: emergeny shut off has prio
  note: Communication loss
  note: 2 nd failure ?
  note: > 1 failure --> fail safe state
  note: double fault prevention
  note: double fault prevention
  note: double fault prevention
  note: fix failure
  note: fix failure
  note: fix failure
  note: fix failure
  note: fix failure
  note: fix failure
  Mvb_stOperModAct : Inport
  ElM_stOperModAct : Inport  Port=2
  Ddc_stOperModAct : Inport  Port=3
  Mvl_stOperModAct : Inport  Port=4
  Eem_stAct : Inport  Port=5
  Add : Sum  Inputs=+++  RndMeth=Simplest  SaturateOnIntegerOverflow=on
  Constant : Constant  Value=200  OutDataTypeStr=OneToOne_U16
  Constant1 : Constant  Value=300  OutDataTypeStr=OneToOne_U16
  Constant{8..11} (4 alike) : Constant  Value=15  OutDataTypeStr=uint8
  Constant12 : Constant  Value=6  OutDataTypeStr=uint8
  Constant13 : Constant  Value=250  OutDataTypeStr=OneToOne_U16
  Constant{14..16,18..20} (6 alike) : Constant  Value=5  OutDataTypeStr=uint8
  Constant17 : Constant  Value=550  OutDataTypeStr=OneToOne_U16
  Constant2 : Constant  Value=400  OutDataTypeStr=OneToOne_U16
  Constant{21..26} (6 alike) : Constant  Value=0  OutDataTypeStr=boolean
  Constant3 : Constant  Value=500  OutDataTypeStr=OneToOne_U16
  Constant4 : Constant  Value=600  OutDataTypeStr=OneToOne_U16
  Constant5 : Constant  Value=700  OutDataTypeStr=OneToOne_U16
  Constant6 : Constant  Value=0  OutDataTypeStr=OneToOne_U16
  Constant7 : Constant  Value=600  OutDataTypeStr=OneToOne_U16
  GetDscPermission : DSM_Library/GetDscPermission  ParFID=FId_MvGridBattDiscnct  ParSimMode=off  ParSimResult=True  Par_SimMode=Simple Simulation  Par_SimRes=TRUE  Par_SimResult=1
  GetDscPermission1 : DSM_Library/GetDscPermission  ParFID=FId_MvGridBRMChrgRed  ParSimMode=off  ParSimResult=True  Par_SimMode=Simple Simulation  Par_SimRes=TRUE  Par_SimResult=1
  GetDscPermission2 : DSM_Library/GetDscPermission  ParFID=FId_MvGridBRMOff  ParSimMode=off  ParSimResult=True  Par_SimMode=Simple Simulation  Par_SimRes=TRUE  Par_SimResult=1
  GetDscPermission3 : DSM_Library/GetDscPermission  ParFID=FId_MvGridDcdcOff  ParSimMode=off  ParSimResult=True  Par_SimMode=Simple Simulation  Par_SimRes=TRUE  Par_SimResult=1
  GetDscPermission4 : DSM_Library/GetDscPermission  ParFID=FId_MvGridBRMBattDcdcOff  ParSimMode=off  ParSimResult=True  Par_SimMode=Simple Simulation  Par_SimRes=TRUE  Par_SimResult=1
  GetDscPermission5 : DSM_Library/GetDscPermission  ParFID=FId_MvGridEmgyOff  ParSimMode=off  ParSimResult=True  Par_SimMode=Simple Simulation  Par_SimRes=TRUE  Par_SimResult=1
  GetDscPermission6 : DSM_Library/GetDscPermission  ParFID=FId_MvGridBattDiscnctComIntrpt  ParSimMode=off  ParSimResult=True  Par_SimMode=Simple Simulation  Par_SimRes=TRUE  Par_SimResult=1
  GetDscPermission8 : DSM_Library/GetDscPermission  ParFID=FId_MvGridDcdcOffComIntrpt  ParSimMode=off  ParSimResult=True  Par_SimMode=Simple Simulation  Par_SimRes=TRUE  Par_SimResult=1
  LogicalOperator : Logic  Operator=OR  Inputs=3  AllPortsSameDT=off  OutDataTypeStr=boolean
  LogicalOperator{1..2,5..6,13} (5 alike) : Logic  Operator=OR  AllPortsSameDT=off  OutDataTypeStr=boolean
  LogicalOperator{3..4,7..12} (8 alike) : Logic  Operator=NOT  AllPortsSameDT=off  OutDataTypeStr=boolean
  LogicalOperator{14..22} (9 alike) : Logic  AllPortsSameDT=off  OutDataTypeStr=boolean
  RSFlipFlop : Efx_Library/Efx_RSFlipFlop  Par_state=Eem_RSFlipFlop550  Par_StateOld=Eem_RSFlipFlop550
      settings: AttributesFormatString=%<Par_State>
  RSFlipFlop1 : Efx_Library/Efx_RSFlipFlop  Par_state=Eem_RSFlipFlop500  Par_StateOld=Eem_RSFlipFlop500
      settings: AttributesFormatString=%<Par_State>
  RSFlipFlop2 : Efx_Library/Efx_RSFlipFlop  Par_state=Eem_RSFlipFlop400  Par_StateOld=Eem_RSFlipFlop400
      settings: AttributesFormatString=%<Par_State>
  RSFlipFlop3 : Efx_Library/Efx_RSFlipFlop  Par_state=Eem_RSFlipFlop300  Par_StateOld=Eem_RSFlipFlop300
      settings: AttributesFormatString=%<Par_State>
  RSFlipFlop4 : Efx_Library/Efx_RSFlipFlop  Par_state=Eem_RSFlipFlop250  Par_StateOld=Eem_RSFlipFlop250
      settings: AttributesFormatString=%<Par_State>
  RSFlipFlop5 : Efx_Library/Efx_RSFlipFlop  Par_state=Eem_RSFlipFlop200  Par_StateOld=Eem_RSFlipFlop200
      settings: AttributesFormatString=%<Par_State>
  RelationalOperator{1..4,12} (5 alike) : RelationalOperator  Operator===  OutDataTypeStr=boolean
  RelationalOperator{5..10} (6 alike) : RelationalOperator  Operator=>  OutDataTypeStr=boolean
  Switch{,1..5,7,9} (8 alike) : Switch  Criteria=u2 ~= 0  RndMeth=Simplest  SaturateOnIntegerOverflow=on
      settings: AttributesFormatString=%<Criteria>\nThreshold:%<Threshold>
  Switch6 : Switch  Criteria=u2 > Threshold  Threshold=1  RndMeth=Simplest  SaturateOnIntegerOverflow=on
      settings: AttributesFormatString=%<Criteria>\nThreshold:%<Threshold>
  Terminator : Terminator
  UnitDelay : UnitDelay  SampleTime=-1
      settings: AttributesFormatString=Init: %<X0>
  Eem_stDesBkup : Outport
  wires:
  ElM_stOperModAct/1 -> RelationalOperator2/1
  Ddc_stOperModAct/1 -> RelationalOperator3/1
  Mvl_stOperModAct/1 -> RelationalOperator4/1
  Mvb_stOperModAct/1 -> RelationalOperator12/1, RelationalOperator1/1
  GetDscPermission/1 -> LogicalOperator7/1
  Constant8/1 -> RelationalOperator1/2
  Constant9/1 -> RelationalOperator2/2
  Constant10/1 -> RelationalOperator3/2
  Constant11/1 -> RelationalOperator4/2
  RelationalOperator1/1 -> LogicalOperator/2
  RelationalOperator2/1 -> LogicalOperator1/2
  GetDscPermission2/1 -> LogicalOperator9/1
  GetDscPermission3/1 -> LogicalOperator10/1
  RelationalOperator3/1 -> LogicalOperator2/2
  RelationalOperator4/1 -> Terminator/1
  GetDscPermission1/1 -> LogicalOperator15/2, LogicalOperator8/1
  GetDscPermission4/1 -> LogicalOperator11/1
  GetDscPermission5/1 -> LogicalOperator12/1
  LogicalOperator12/1 -> Switch5/2
  LogicalOperator10/1 -> LogicalOperator2/1
  LogicalOperator9/1 -> LogicalOperator1/1
  LogicalOperator7/1 -> LogicalOperator/1
  Constant7/1 -> Switch6/1
  Constant6/1 -> Switch/3
  Constant/1 -> Switch/1
  Constant1/1 -> Switch1/1
  Switch4/1 -> Switch6/3
  Constant2/1 -> Switch2/1
  Constant3/1 -> Switch3/1
  Constant4/1 -> Switch4/1
  Constant5/1 -> Switch5/1
  Constant12/1 -> RelationalOperator12/2
  RelationalOperator12/1 -> LogicalOperator/3
  Constant13/1 -> Switch7/1
  Constant17/1 -> Switch9/1
  GetDscPermission6/1 -> LogicalOperator14/1, LogicalOperator3/1
  GetDscPermission8/1 -> LogicalOperator16/1, LogicalOperator4/1
  Switch/1 -> Switch7/3
  Switch7/1 -> Switch1/3
  Switch1/1 -> Switch2/3
  Switch2/1 -> Switch3/3
  LogicalOperator2/1 -> LogicalOperator16/2
  Switch3/1 -> Switch9/3
  Switch9/1 -> Switch4/3
  LogicalOperator11/1 -> Switch4/2
  Switch6/1 -> Switch5/3
  Switch5/1 -> Eem_stDesBkup/1
  Add/1 -> Switch6/2
  RSFlipFlop1/1 -> LogicalOperator13/2, Switch3/2
  RSFlipFlop3/1 -> LogicalOperator6/2, Switch1/2
  RSFlipFlop2/1 -> LogicalOperator6/1, Switch2/2
  RSFlipFlop5/1 -> LogicalOperator5/2, Switch/2
  RSFlipFlop4/1 -> LogicalOperator5/1, Switch7/2
  Constant21/1 -> RSFlipFlop/1
  RSFlipFlop/1 -> LogicalOperator13/1, Switch9/2
  Constant22/1 -> RSFlipFlop1/1
  LogicalOperator4/1 -> LogicalOperator22/2
  Constant23/1 -> RSFlipFlop2/1
  Constant24/1 -> RSFlipFlop3/1
  Constant25/1 -> RSFlipFlop4/1
  Constant26/1 -> RSFlipFlop5/1
  LogicalOperator6/1 -> Add/2
  LogicalOperator5/1 -> Add/3
  LogicalOperator13/1 -> Add/1
  LogicalOperator/1 -> LogicalOperator14/2
  LogicalOperator1/1 -> LogicalOperator15/1
  LogicalOperator15/1 -> LogicalOperator20/2
  LogicalOperator16/1 -> LogicalOperator21/2
  Constant14/1 -> RelationalOperator5/2
  RelationalOperator5/1 -> LogicalOperator17/1
  LogicalOperator3/1 -> LogicalOperator17/2
  LogicalOperator17/1 -> RSFlipFlop4/2
  Constant15/1 -> RelationalOperator6/2
  RelationalOperator6/1 -> LogicalOperator18/1
  LogicalOperator14/1 -> LogicalOperator18/2
  LogicalOperator18/1 -> RSFlipFlop5/2
  Constant16/1 -> RelationalOperator7/2
  RelationalOperator7/1 -> LogicalOperator19/1
  LogicalOperator8/1 -> LogicalOperator19/2
  LogicalOperator19/1 -> RSFlipFlop3/2
  Constant18/1 -> RelationalOperator8/2
  RelationalOperator8/1 -> LogicalOperator20/1
  LogicalOperator20/1 -> RSFlipFlop2/2
  Constant19/1 -> RelationalOperator9/2
  Eem_stAct/1 -> UnitDelay/1
  RelationalOperator9/1 -> LogicalOperator21/1
  LogicalOperator21/1 -> RSFlipFlop1/2
  Constant20/1 -> RelationalOperator10/2
  RelationalOperator10/1 -> LogicalOperator22/1
  LogicalOperator22/1 -> RSFlipFlop/2
  UnitDelay/1 -> RelationalOperator5/1, RelationalOperator6/1, RelationalOperator10/1, RelationalOperator9/1, RelationalOperator8/1, RelationalOperator7/1

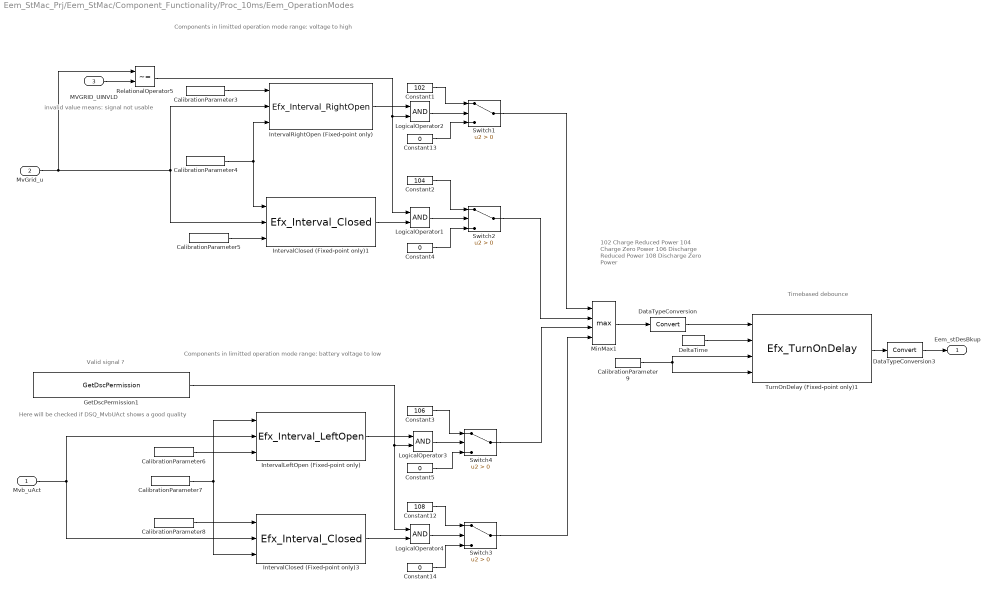
== system Eem_StMac_Prj/Eem_StMac/Component_Functionality/Proc_10ms/Eem_OperationModes ==
  note: invalid value means: signal not usable
  note: Timebased debounce
  note: 102  Charge Reduced Power
      | 104  Charge Zero Power
      | 106  Discharge Reduced Power
      | 108  Discharge Zero Power
  note: Components in limitted operation mode range: battery voltage to low
  note: Components in limitted operation mode range: voltage to high
  note: Valid signal ?
  note: Here will be checked if DSQ_MvbUAct shows a good quality
  Mvb_uAct : Inport
  MvGrid_u : Inport  Port=2  OutDataTypeStr=spg_q0p0039_S16
  MVGRID_UINVLD : Inport  Port=3
  CalibrationParameter3 : Parameter_Lib/CalibrationParameter  ParName=Eem_uLim1MvGrid_C  ParVal=52  ParValStruct=<1x1 struct>  ParValDt=spg_q0p0039_S16  Par_MDX=off  ParNameOld=Eem_uLim1MvGrid_C  Value=0  Par_Name=0
      settings: AttributesFormatString=%<ParName>
  CalibrationParameter4 : Parameter_Lib/CalibrationParameter  ParName=Eem_uLim2MvGrid_C  ParVal=54  ParValStruct=<1x1 struct>  ParValDt=spg_q0p0039_S16  Par_MDX=off  ParNameOld=Eem_uLim2MvGrid_C  Value=0  Par_Name=0
      settings: AttributesFormatString=%<ParName>
  CalibrationParameter5 : Parameter_Lib/CalibrationParameter  ParName=Eem_uLim3MvGrid_C  ParVal=127  ParValStruct=<1x1 struct>  ParValDt=spg_q0p0039_S16  Par_MDX=off  ParNameOld=Eem_uLim3MvGrid_C  Value=0  Par_Name=0
      settings: AttributesFormatString=%<ParName>
  CalibrationParameter6 : Parameter_Lib/CalibrationParameter  ParName=Eem_uLim1Mvb_C  ParVal=36  ParValStruct=<1x1 struct>  ParValDt=spg_q0p0039_S16  Par_MDX=off  ParNameOld=Eem_uLim1Mvb_C  Value=0  Par_Name=0
      settings: AttributesFormatString=%<ParName>
  CalibrationParameter7 : Parameter_Lib/CalibrationParameter  ParName=Eem_uLim2Mvb_C  ParVal=30  ParValStruct=<1x1 struct>  ParValDt=spg_q0p0039_S16  Par_MDX=off  ParNameOld=Eem_uLim2Mvb_C  Value=0  Par_Name=0
      settings: AttributesFormatString=%<ParName>
  CalibrationParameter8 : Parameter_Lib/CalibrationParameter  ParName=Eem_uLim3Mvb_C  ParVal=1  ParValStruct=<1x1 struct>  ParValDt=spg_q0p0039_S16  Par_MDX=off  ParNameOld=Eem_uLim3Mvb_C  Value=0  Par_Name=0
      settings: AttributesFormatString=%<ParName>
  CalibrationParameter9 : Parameter_Lib/CalibrationParameter  ParName=Eem_tiDebTmpRstrcn_C  ParVal=10  ParValStruct=<1x1 struct>  ParValDt=RBPtCel_ti_0p01_1_S16  Par_MDX=off  ParNameOld=Eem_tiDebTmpRstrcn_C  Value=0  Par_Name=0
      settings: AttributesFormatString=%<ParName>
  Constant1 : Constant  Value=102  OutDataTypeStr=OneToOne_U16
  Constant12 : Constant  Value=108  OutDataTypeStr=OneToOne_U16
  Constant{4..5,13..14} (4 alike) : Constant  Value=0  OutDataTypeStr=OneToOne_U16
  Constant2 : Constant  Value=104  OutDataTypeStr=OneToOne_U16
  Constant3 : Constant  Value=106  OutDataTypeStr=OneToOne_U16
  DataTypeConversion : DataTypeConversion  RndMeth=Simplest  SaturateOnIntegerOverflow=on
  DataTypeConversion3 : DataTypeConversion  RndMeth=Simplest  SaturateOnIntegerOverflow=on
  DeltaTime : DeltaTime_Lib/DeltaTime  outDType=sfix32_S1en6  initVal=.01
  GetDscPermission1 : DSM_Library/GetDscPermission  ParFID=FId_StMacDisChrgRed  ParSimMode=off  ParSimResult=True  Par_SimMode=Simple Simulation  Par_SimRes=TRUE  Par_SimResult=1
  IntervalClosed (Fixed-point only)1 : Efx_Library/Efx_Interval_Closed
  IntervalClosed (Fixed-point only)3 : Efx_Library/Efx_Interval_Closed
  IntervalLeftOpen (Fixed-point only) : Efx_Library/Efx_Interval_LeftOpen
  IntervalRightOpen (Fixed-point only) : Efx_Library/Efx_Interval_RightOpen
  LogicalOperator{1..4} (4 alike) : Logic  AllPortsSameDT=off  OutDataTypeStr=boolean
  MinMax1 : MinMax  Function=max  Inputs=4  OutDataTypeStr=OneToOne_U16  RndMeth=Simplest  SaturateOnIntegerOverflow=on
  RelationalOperator5 : RelationalOperator  Operator=~=  OutDataTypeStr=boolean
  Switch{1..4} (4 alike) : Switch  Criteria=u2 > Threshold  RndMeth=Simplest  SaturateOnIntegerOverflow=on
      settings: AttributesFormatString=%<Criteria>\nThreshold:%<Threshold>
  TurnOnDelay (Fixed-point only)1 : Efx_Library/Efx_TurnOnDelay  Par_Mode=Calculation  Par_State=Eem_Debounce  Par_Deb=on  Par_TrnOn=off  Par_TrnOff=off  Par_StateOld=Eem_Debounce
      settings: AttributesFormatString=%<Par_State>
  Eem_stDesBkup : Outport  OutDataTypeStr=OneToOne_U16
  wires:
  MvGrid_u/1 -> RelationalOperator5/1, IntervalRightOpen (Fixed-point only)/2, IntervalClosed (Fixed-point only)1/2
  Constant1/1 -> Switch1/1
  Constant13/1 -> Switch1/3
  Constant2/1 -> Switch2/1
  Constant4/1 -> Switch2/3
  Constant3/1 -> Switch4/1
  Constant5/1 -> Switch4/3
  Constant12/1 -> Switch3/1
  Constant14/1 -> Switch3/3
  Switch1/1 -> MinMax1/1
  Switch2/1 -> MinMax1/2
  Switch4/1 -> MinMax1/3
  Switch3/1 -> MinMax1/4
  CalibrationParameter3/1 -> IntervalRightOpen (Fixed-point only)/1
  CalibrationParameter4/1 -> IntervalRightOpen (Fixed-point only)/3, IntervalClosed (Fixed-point only)1/1
  CalibrationParameter7/1 -> IntervalLeftOpen (Fixed-point only)/1, IntervalClosed (Fixed-point only)3/3
  CalibrationParameter5/1 -> IntervalClosed (Fixed-point only)1/3
  CalibrationParameter6/1 -> IntervalLeftOpen (Fixed-point only)/3
  CalibrationParameter8/1 -> IntervalClosed (Fixed-point only)3/1
  Mvb_uAct/1 -> IntervalLeftOpen (Fixed-point only)/2, IntervalClosed (Fixed-point only)3/2
  IntervalRightOpen (Fixed-point only)/1 -> LogicalOperator2/1
  LogicalOperator2/1 -> Switch1/2
  LogicalOperator1/1 -> Switch2/2
  IntervalClosed (Fixed-point only)1/1 -> LogicalOperator1/2
  IntervalLeftOpen (Fixed-point only)/1 -> LogicalOperator3/1
  GetDscPermission1/1 -> LogicalOperator4/1, LogicalOperator3/2
  LogicalOperator3/1 -> Switch4/2
  IntervalClosed (Fixed-point only)3/1 -> LogicalOperator4/2
  LogicalOperator4/1 -> Switch3/2
  MVGRID_UINVLD/1 -> RelationalOperator5/2
  RelationalOperator5/1 -> LogicalOperator1/1, LogicalOperator2/2
  DeltaTime/1 -> TurnOnDelay (Fixed-point only)1/2
  DataTypeConversion3/1 -> Eem_stDesBkup/1
  DataTypeConversion/1 -> TurnOnDelay (Fixed-point only)1/1
  TurnOnDelay (Fixed-point only)1/1 -> DataTypeConversion3/1
  MinMax1/1 -> DataTypeConversion/1
  CalibrationParameter9/1 -> TurnOnDelay (Fixed-point only)1/3, TurnOnDelay (Fixed-point only)1/4

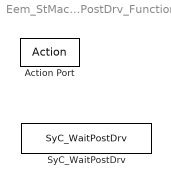
== system Eem_StMac_Prj/Eem_StMac/Component_Functionality/Proc_10ms/SyC_WaitPostDrv_Function ==
  Action Port : ActionPort  ActionType=then
      settings: AttributesFormatString=%<InitializeStates>
  SyC_WaitPostDrv : SYC_Library/SyC_WaitPostDrv

== stateflow chart Eem_StMac_Prj/Scheduler/Chart1 ==
  settings: executeAtInitialization=1
  state Ini [parallel]
    settings: executionOrder=1
    Ini -> Ini : [isIni]{Ini_Task; isIni=false;}
  state T0001 [parallel]
    on every(1,tic): ESC_tiSampling_s=0.001;
    on every(1,tic): ASync_dT=ASync_dT+0.001;
    on every(1,tic): Task_1ms;
    settings: executionOrder=2
  state T0002 [parallel]
    on every(2,tic): ESC_tiSampling_s=0.002;
    on every(2,tic): Task_2ms;
    settings: executionOrder=3
  state T0005 [parallel]
    on every(5,tic): ESC_tiSampling_s=0.005;
    on every(5,tic): Task_5ms;
    settings: executionOrder=4
  state T0010 [parallel]
    on every(10,tic): ESC_tiSampling_s=0.01;
    on every(10,tic): Task_10ms;
    settings: executionOrder=5
  state T0020 [parallel]
    on every(20,tic): ESC_tiSampling_s=0.02;
    on every(20,tic): Task_20ms;
    settings: executionOrder=6
  state T0050 [parallel]
    on every(50,tic): ESC_tiSampling_s=0.05;
    on every(50,tic): Task_50ms;
    settings: executionOrder=7
  state T0100 [parallel]
    on every(100,tic): ESC_tiSampling_s=0.1;
    on every(100,tic): Task_100ms;
    settings: executionOrder=8
  state T0200 [parallel]
    on every(200,tic): ESC_tiSampling_s=0.2;
    on every(200,tic): Task_200ms;
    settings: executionOrder=9
  state T1000 [parallel]
    on every(1000,tic): ESC_tiSampling_s=1;
    on every(1000,tic): Task_1000ms;
    settings: executionOrder=10
  state ASync [parallel]
    settings: executionOrder=11
    ASync -> ASync : [ASync_U!=0]{ESC_tiSampling_s=ASync_dT;ASync_Task;ASync_dT=0;}
  (default) -> Ini
  data: isIni local double =true; ASync_U input uint8; ESC_tiSampling_s output fixdt(1,32,1.0e-6,0); ASync_dT local fixdt(1,32,1.0e-6,0) =0
  events: Task_1ms output FUNCTION_CALL_EVENT; Task_2ms output FUNCTION_CALL_EVENT; Task_5ms output FUNCTION_CALL_EVENT; Task_10ms output FUNCTION_CALL_EVENT; Task_20ms output FUNCTION_CALL_EVENT; Task_50ms output FUNCTION_CALL_EVENT; Task_100ms output FUNCTION_CALL_EVENT; Task_200ms output FUNCTION_CALL_EVENT; Task_1000ms output FUNCTION_CALL_EVENT; Ini_Task output FUNCTION_CALL_EVENT; ASync_Task output FUNCTION_CALL_EVENT; tic input EITHER_EDGE_EVENT
